simulink model "threeDOF_PDcontrol17"  (R2017b)
settings: Solver=VariableStepAuto  StartTime=0.0  StopTime=15  RelTol=1e-3
model workspace (MAT data in the model file):
  D = 1
  K = 4
  m = 2
  v0 = [0 0 0]
  x0 = [10 15 20]
  x_des = [5 5 5]
settings Model: Creator=Tommaso  LastModifiedBy=Tommaso
settings DataIOCC: ReturnWorkspaceOutputs=on
settings DebuggingCC: UnconnectedInputMsg=none  UnconnectedOutputMsg=none  UnconnectedLineMsg=none  SFMachineParentedDataDiag=error
settings SFSimCC: SimUseLocalCustomCode=on
settings RTWCC: RTWUseLocalCustomCode=on

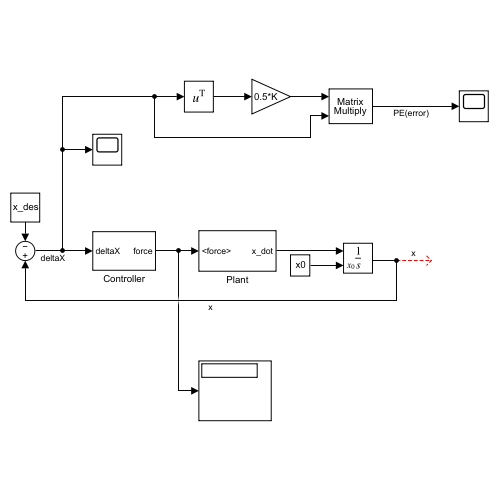
[thumbnail: Simulink's stored preview of the top-level diagram]
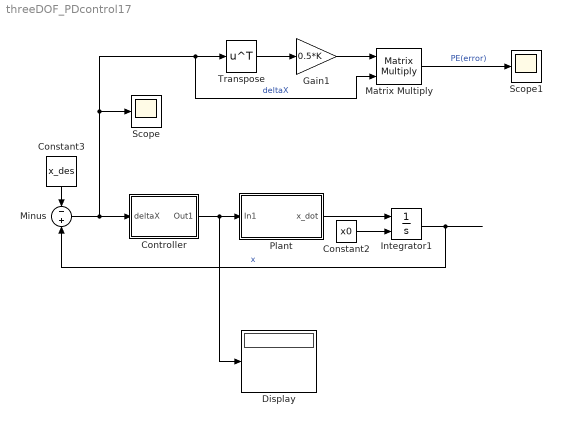
== system threeDOF_PDcontrol17 ==
  Constant2 : Constant  Value=x0
  Constant3 : Constant  Value=x_des
  Controller : Subsystem
  Display : Display
  Gain1 : Gain  Gain=0.5*K
  Integrator1 : Integrator  InitialConditionSource=external
  Matrix Multiply : Product  Multiplication=Matrix(*)
  Minus : Sum  Inputs=-+
  Plant : Subsystem
  Scope : Scope
  Scope1 : Scope
  Transpose : Math  Operator=transpose  SaturateOnIntegerOverflow=on
  wires:
  Transpose/1 -> Gain1/1
  Constant3/1 -> Minus/1
  Gain1/1 -> Matrix Multiply/1
  Minus/1 -> Controller/1(deltaX), Matrix Multiply/2, Transpose/1, Scope/1  "deltaX"
  Integrator1/1 -> Minus/2  "x"
  Constant2/1 -> Integrator1/2
  Controller/1(Out1) -> Display/1, Plant/1(In1)
  Plant/1(x_dot) -> Integrator1/1
  Matrix Multiply/1 -> Scope1/1  "PE(error)"

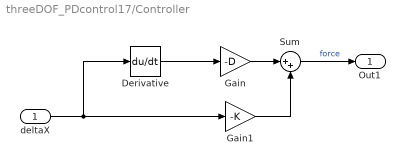
== system threeDOF_PDcontrol17/Controller ==
  deltaX : Inport
  Derivative : Derivative
  Gain : Gain  Gain=-D
  Gain1 : Gain  Gain=-K
  Sum : Sum  Inputs=|++
  Out1 : Outport
  wires:
  deltaX/1 -> Derivative/1, Gain1/1
  Gain/1 -> Sum/1
  Gain1/1 -> Sum/2
  Sum/1 -> Out1/1  "force"
  Derivative/1 -> Gain/1

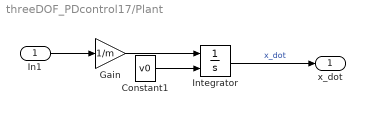
== system threeDOF_PDcontrol17/Plant ==
  In1 : Inport
  Constant1 : Constant  Value=v0
  Gain : Gain  Gain=1/m
  Integrator : Integrator  InitialConditionSource=external
  x_dot : Outport
  wires:
  Gain/1 -> Integrator/1
  Constant1/1 -> Integrator/2
  Integrator/1 -> x_dot/1  "x_dot"
  In1/1 -> Gain/1
